simulink model "SwarmGeomagneticHarness"  (R2025a)
settings: Solver=ode45  StartTime=0  StopTime=200  RelTol=1e-09  AbsTol=1e-10
settings Model: Creator=aocs-simulation  LastModifiedBy=juliankazmierski

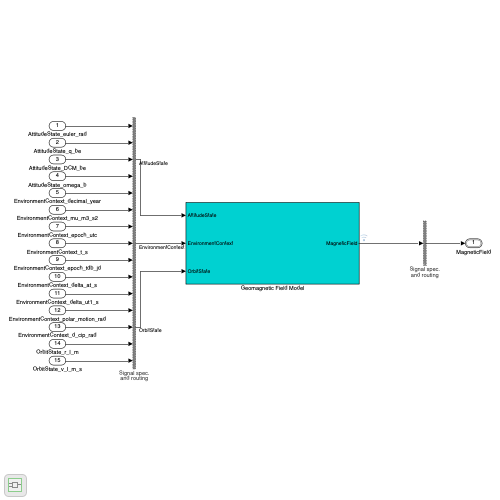
[thumbnail: Simulink's stored preview of the top-level diagram]
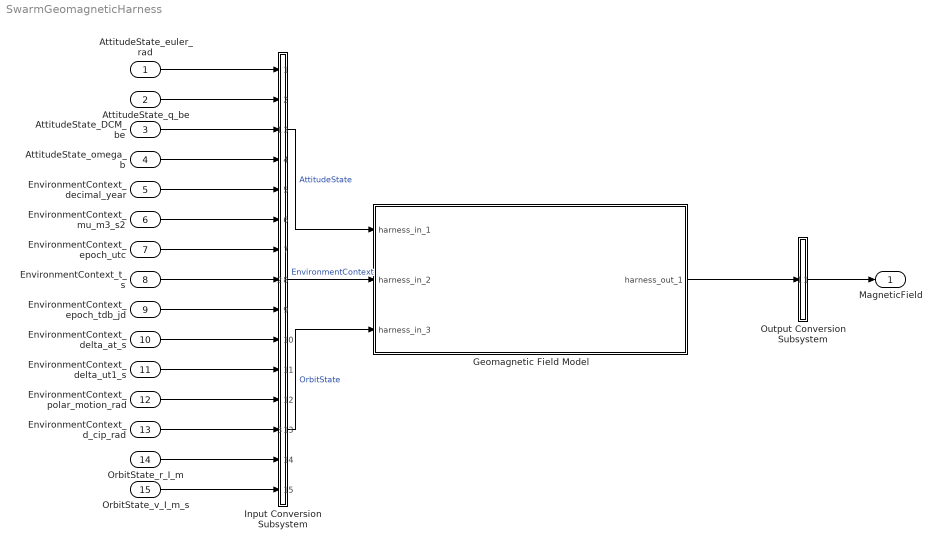
== system SwarmGeomagneticHarness ==
  AttitudeState_euler_rad : Inport  OutDataTypeStr=double  PortDimensions=[3]  SampleTime=0
  AttitudeState_q_be : Inport  Port=2  OutDataTypeStr=double  PortDimensions=[4]  SampleTime=0
  AttitudeState_DCM_be : Inport  Port=3  OutDataTypeStr=double  PortDimensions=[3, 3]  SampleTime=0
  AttitudeState_omega_b : Inport  Port=4  OutDataTypeStr=double  PortDimensions=[3]  SampleTime=0
  EnvironmentContext_decimal_year : Inport  Port=5  OutDataTypeStr=double  PortDimensions=[1]  SampleTime=0
  EnvironmentContext_mu_m3_s2 : Inport  Port=6  OutDataTypeStr=double  PortDimensions=[1, 1]  SampleTime=[-1, 0]
  EnvironmentContext_epoch_utc : Inport  Port=7  OutDataTypeStr=double  PortDimensions=[6, 1]  SampleTime=[-1, 0]
  EnvironmentContext_t_s : Inport  Port=8  OutDataTypeStr=double  PortDimensions=[1]  SampleTime=0
  EnvironmentContext_epoch_tdb_jd : Inport  Port=9  OutDataTypeStr=double  PortDimensions=[1, 1]  SampleTime=[-1, 0]
  EnvironmentContext_delta_at_s : Inport  Port=10  OutDataTypeStr=double  PortDimensions=[1]  SampleTime=[-1, 0]
  EnvironmentContext_delta_ut1_s : Inport  Port=11  OutDataTypeStr=double  PortDimensions=[1]  SampleTime=[-1, 0]
  EnvironmentContext_polar_motion_rad : Inport  Port=12  OutDataTypeStr=double  PortDimensions=[2]  SampleTime=[-1, 0]
  EnvironmentContext_d_cip_rad : Inport  Port=13  OutDataTypeStr=double  PortDimensions=[2]  SampleTime=[-1, 0]
  OrbitState_r_I_m : Inport  Port=14  OutDataTypeStr=double  PortDimensions=[3]  SampleTime=0
  OrbitState_v_I_m_s : Inport  Port=15  OutDataTypeStr=double  PortDimensions=[3]  SampleTime=0
  Geomagnetic Field Model : Subsystem  Tag=__SL_testing_harness_stub_
  Input Conversion Subsystem : Subsystem  Tag=__SLT_ICS__  Description=|
      | Signal spec.
      | and routing
      settings: AttributesFormatString=%<Description>
  Output Conversion Subsystem : Subsystem  Tag=__SLT_OCS__  Description=|
      | Signal spec.
      | and routing
      settings: AttributesFormatString=%<Description>
  MagneticField : Outport  OutDataTypeStr=Bus: MagneticFieldBus
  wires:
  AttitudeState_euler_rad/1 -> Input Conversion Subsystem/1(Inport_1)
  AttitudeState_q_be/1 -> Input Conversion Subsystem/2(Inport_2)
  AttitudeState_DCM_be/1 -> Input Conversion Subsystem/3(Inport_3)
  AttitudeState_omega_b/1 -> Input Conversion Subsystem/4(Inport_4)
  EnvironmentContext_decimal_year/1 -> Input Conversion Subsystem/5(Inport_5)
  EnvironmentContext_mu_m3_s2/1 -> Input Conversion Subsystem/6(Inport_6)
  EnvironmentContext_epoch_utc/1 -> Input Conversion Subsystem/7(Inport_7)
  EnvironmentContext_t_s/1 -> Input Conversion Subsystem/8(Inport_8)
  EnvironmentContext_epoch_tdb_jd/1 -> Input Conversion Subsystem/9(Inport_9)
  EnvironmentContext_delta_at_s/1 -> Input Conversion Subsystem/10(Inport_10)
  EnvironmentContext_delta_ut1_s/1 -> Input Conversion Subsystem/11(Inport_11)
  EnvironmentContext_polar_motion_rad/1 -> Input Conversion Subsystem/12(Inport_12)
  EnvironmentContext_d_cip_rad/1 -> Input Conversion Subsystem/13(Inport_13)
  OrbitState_r_I_m/1 -> Input Conversion Subsystem/14(Inport_14)
  OrbitState_v_I_m_s/1 -> Input Conversion Subsystem/15(Inport_15)
  Output Conversion Subsystem/1(Outport_1) -> MagneticField/1
  Input Conversion Subsystem/1(Outport_1) -> Geomagnetic Field Model/1(harness_in_1)  "AttitudeState"
  Input Conversion Subsystem/2(Outport_2) -> Geomagnetic Field Model/2(harness_in_2)  "EnvironmentContext"
  Input Conversion Subsystem/3(Outport_3) -> Geomagnetic Field Model/3(harness_in_3)  "OrbitState"
  Geomagnetic Field Model/1(harness_out_1) -> Output Conversion Subsystem/1(Inport_1)

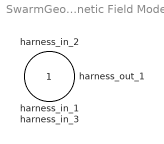
== system SwarmGeomagneticHarness/Geomagnetic Field Model ==
  harness_in_1 : Inport
  harness_in_2 : Inport  Port=2
  harness_in_3 : Inport  Port=3
  harness_out_1 : Outport

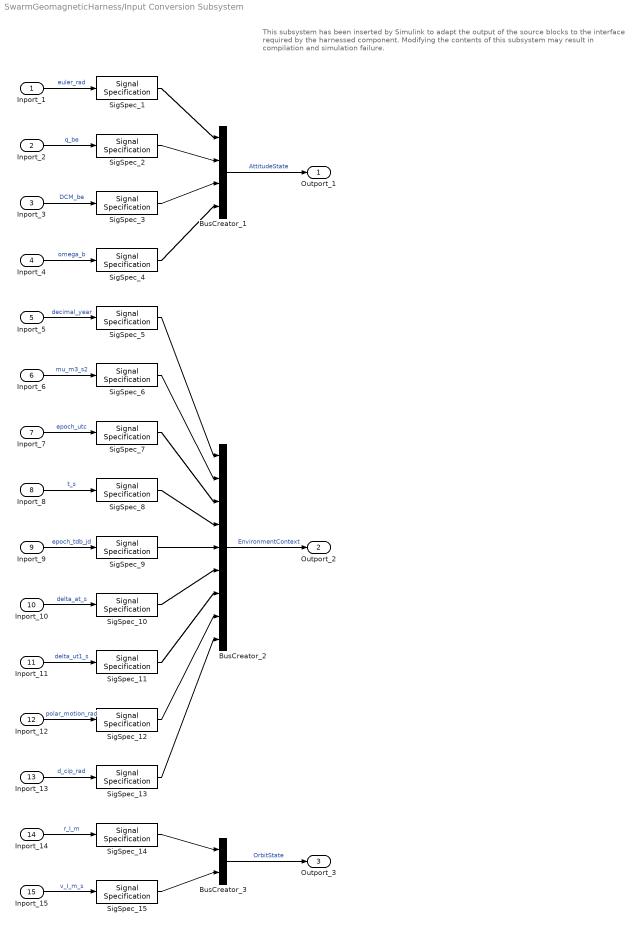
== system SwarmGeomagneticHarness/Input Conversion Subsystem ==
  note: This subsystem has been inserted by Simulink to adapt the output of the source blocks to the interface required by the harnessed component.
      |  Modifying the contents of this subsystem may result in compilation and simulation failure.
  Inport_1 : Inport
  Inport_2 : Inport  Port=2
  Inport_3 : Inport  Port=3
  Inport_4 : Inport  Port=4
  Inport_5 : Inport  Port=5
  Inport_6 : Inport  Port=6
  Inport_7 : Inport  Port=7
  Inport_8 : Inport  Port=8
  Inport_9 : Inport  Port=9
  Inport_10 : Inport  Port=10
  Inport_11 : Inport  Port=11
  Inport_12 : Inport  Port=12
  Inport_13 : Inport  Port=13
  Inport_14 : Inport  Port=14
  Inport_15 : Inport  Port=15
  BusCreator_1 : BusCreator  Inputs=4
  BusCreator_2 : BusCreator  Inputs=9  OutDataTypeStr=Bus: EnvironmentContextBus
  BusCreator_3 : BusCreator  Inputs=2
  SigSpec_1 : SignalSpecification  OutDataTypeStr=double  Unit=rad  Dimensions=[3]  SampleTime=[0, 0]
  SigSpec_10 : SignalSpecification  OutDataTypeStr=double  Unit=sec  Dimensions=[1]  SampleTime=[-1, 0]
  SigSpec_11 : SignalSpecification  OutDataTypeStr=double  Unit=sec  Dimensions=[1]  SampleTime=[-1, 0]
  SigSpec_12 : SignalSpecification  OutDataTypeStr=double  Unit=rad  Dimensions=[2]  SampleTime=[-1, 0]
  SigSpec_13 : SignalSpecification  OutDataTypeStr=double  Unit=rad  Dimensions=[2]  SampleTime=[-1, 0]
  SigSpec_14 : SignalSpecification  OutDataTypeStr=double  Unit=m  Dimensions=[3]  SampleTime=[0, 0]
  SigSpec_15 : SignalSpecification  OutDataTypeStr=double  Unit=m/s  Dimensions=[3]  SampleTime=[0, 0]
  SigSpec_2 : SignalSpecification  OutDataTypeStr=double  Unit=1  Dimensions=[4]  SampleTime=[0, 0]
  SigSpec_3 : SignalSpecification  OutDataTypeStr=double  Unit=1  Dimensions=[3, 3]  SampleTime=[0, 0]
  SigSpec_4 : SignalSpecification  OutDataTypeStr=double  Unit=rad/s  Dimensions=[3]  SampleTime=[0, 0]
  SigSpec_5 : SignalSpecification  OutDataTypeStr=double  Dimensions=[1]  SampleTime=[0, 0]
  SigSpec_6 : SignalSpecification  OutDataTypeStr=double  Unit=m^3/s^2  Dimensions=[1, 1]  SampleTime=[-1, 0]
  SigSpec_7 : SignalSpecification  OutDataTypeStr=double  Unit=1  Dimensions=[6, 1]  SampleTime=[-1, 0]
  SigSpec_8 : SignalSpecification  OutDataTypeStr=double  Dimensions=[1]  SampleTime=[0, 0]
  SigSpec_9 : SignalSpecification  OutDataTypeStr=double  Unit=1  Dimensions=[1, 1]  SampleTime=[-1, 0]
  Outport_1 : Outport
  Outport_2 : Outport  Port=2
  Outport_3 : Outport  Port=3
  wires:
  BusCreator_1/1 -> Outport_1/1  "AttitudeState"
  SigSpec_1/1 -> BusCreator_1/1
  Inport_1/1 -> SigSpec_1/1  "euler_rad"
  SigSpec_2/1 -> BusCreator_1/2
  Inport_2/1 -> SigSpec_2/1  "q_be"
  SigSpec_3/1 -> BusCreator_1/3
  Inport_3/1 -> SigSpec_3/1  "DCM_be"
  SigSpec_4/1 -> BusCreator_1/4
  Inport_4/1 -> SigSpec_4/1  "omega_b"
  BusCreator_2/1 -> Outport_2/1  "EnvironmentContext"
  SigSpec_5/1 -> BusCreator_2/1
  Inport_5/1 -> SigSpec_5/1  "decimal_year"
  SigSpec_6/1 -> BusCreator_2/2
  Inport_6/1 -> SigSpec_6/1  "mu_m3_s2"
  SigSpec_7/1 -> BusCreator_2/3
  Inport_7/1 -> SigSpec_7/1  "epoch_utc"
  SigSpec_8/1 -> BusCreator_2/4
  Inport_8/1 -> SigSpec_8/1  "t_s"
  SigSpec_9/1 -> BusCreator_2/5
  Inport_9/1 -> SigSpec_9/1  "epoch_tdb_jd"
  SigSpec_10/1 -> BusCreator_2/6
  Inport_10/1 -> SigSpec_10/1  "delta_at_s"
  SigSpec_11/1 -> BusCreator_2/7
  Inport_11/1 -> SigSpec_11/1  "delta_ut1_s"
  SigSpec_12/1 -> BusCreator_2/8
  Inport_12/1 -> SigSpec_12/1  "polar_motion_rad"
  SigSpec_13/1 -> BusCreator_2/9
  Inport_13/1 -> SigSpec_13/1  "d_cip_rad"
  BusCreator_3/1 -> Outport_3/1  "OrbitState"
  SigSpec_14/1 -> BusCreator_3/1
  Inport_14/1 -> SigSpec_14/1  "r_I_m"
  SigSpec_15/1 -> BusCreator_3/2
  Inport_15/1 -> SigSpec_15/1  "v_I_m_s"

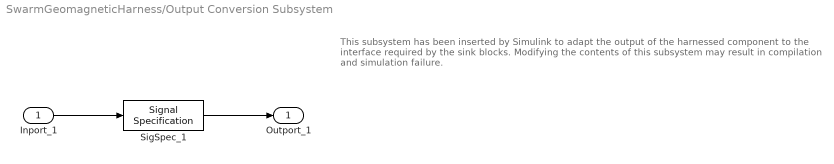
== system SwarmGeomagneticHarness/Output Conversion Subsystem ==
  note: This subsystem has been inserted by Simulink to adapt the output of the harnessed component to the interface required by the sink blocks.
      |  Modifying the contents of this subsystem may result in compilation and simulation failure.
  Inport_1 : Inport
  SigSpec_1 : SignalSpecification  Dimensions=[-1]
  Outport_1 : Outport
  wires:
  Inport_1/1 -> SigSpec_1/1
  SigSpec_1/1 -> Outport_1/1
